simulink model "exercise5s"  (R2025b)
settings: Solver=VariableStepAuto  StartTime=0.0  StopTime=0.01  RelTol=1e-3
values from neighbouring files (symbols this model uses):
  cm = 23.4e-3    (= 0.0234)    [exercise5.m]
  D = 0.4191e-5    (= 4.191e-06)    [exercise5.m]
  J = 0.23e-6    (= 2.3e-07)    [exercise5.m]
  L = 0.23e-3    (= 0.00023)    [exercise5.m]
  R = 2.4    [exercise5.m]
libraries: cstblocks x2
settings Model: Creator=Lenovo  LastModifiedBy=Lenovo

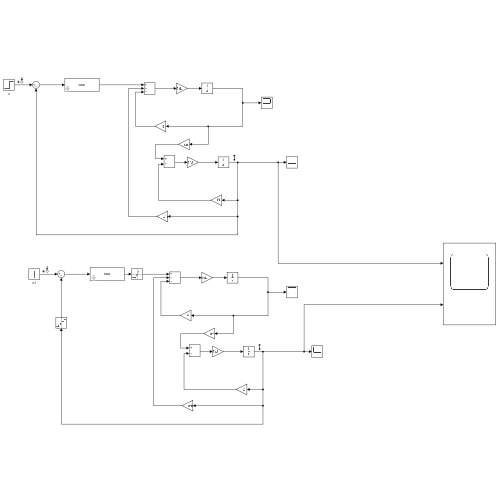
[thumbnail: Simulink's stored preview of the top-level diagram]
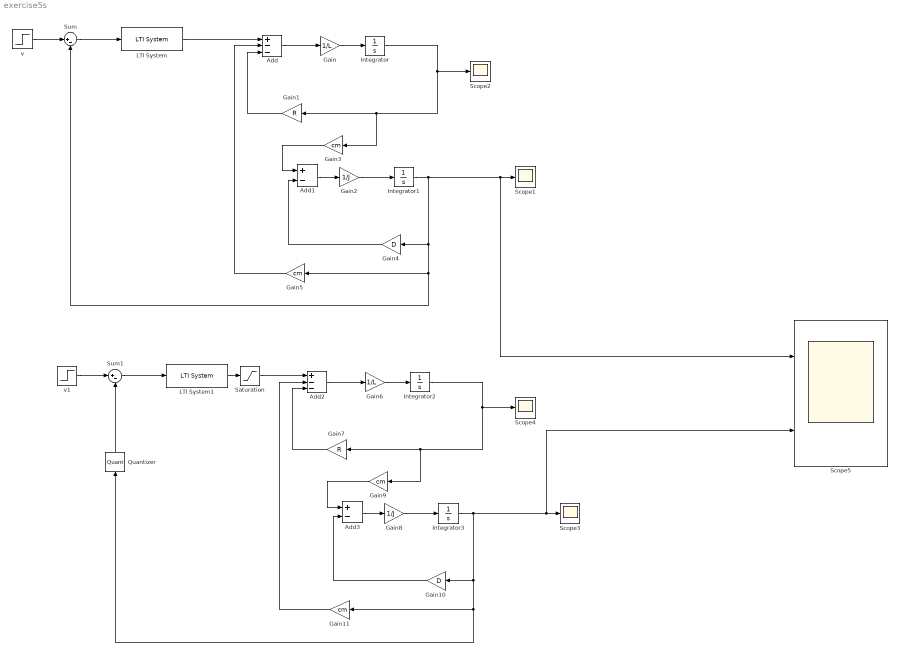
== system exercise5s ==
  Add : Sum  Inputs=+--
  Add1 : Sum  Inputs=+-
  Add2 : Sum  Inputs=+--
  Add3 : Sum  Inputs=+-
  Gain : Gain  Gain=1/L
  Gain1 : Gain  Gain=R
  Gain10 : Gain  Gain=D
  Gain{3,5,9,11} (4 alike) : Gain  Gain=cm
  Gain2 : Gain  Gain=1/J
  Gain4 : Gain  Gain=D
  Gain6 : Gain  Gain=1/L
  Gain7 : Gain  Gain=R
  Gain8 : Gain  Gain=1/J
  Integrator{,1..3} (4 alike) : Integrator
  LTI System : cstblocks/LTI System  sys=cwe  IC=[]  PadeOrder=0
  LTI System1 : cstblocks/LTI System  sys=cwe  IC=[]  PadeOrder=0
  Quantizer : Quantizer  QuantizationInterval=5
  Saturation : Saturate  UpperLimit=12  LowerLimit=-12
  Scope{1..4} (4 alike) : Scope
      Scope1 settings: ActiveDisplayYMinimum=-1  ActiveDisplayYMaximum=1  DataLoggingVariableName=cx
      Scope2 settings: ActiveDisplayYMinimum=-1  ActiveDisplayYMaximum=1  DataLoggingVariableName=cx1
      Scope3 settings: ActiveDisplayYMinimum=-1  ActiveDisplayYMaximum=1  DataLoggingVariableName=cx2
      Scope4 settings: ActiveDisplayYMinimum=-1  ActiveDisplayYMaximum=1  DataLoggingVariableName=cx3
  Scope5 : Scope  NumInputPorts=2
      settings: ActiveDisplayYMinimum=-39.982641044821122  ActiveDisplayYMaximum=359.84376940339018  DataLoggingVariableName=ex5
  Sum : Sum  Inputs=|+-
  Sum1 : Sum  Inputs=|+-
  v : Step  Time=0.001  After=3000*2*3.14/60  SampleTime=0
  v1 : Step  Time=0.001  After=3000*2*3.14/60  SampleTime=0
  wires:
  Gain/1 -> Integrator/1
  Gain3/1 -> Add1/1
  Gain4/1 -> Add1/2
  Add1/1 -> Gain2/1
  Integrator/1 -> Scope2/1, Gain3/1, Gain1/1
  Gain5/1 -> Add/2
  Gain2/1 -> Integrator1/1
  Gain1/1 -> Add/3
  Add/1 -> Gain/1
  Integrator1/1 -> Gain5/1, Sum/2, Gain4/1, Scope5/1, Scope1/1
  Sum/1 -> LTI System/1
  LTI System/1 -> Add/1
  v/1 -> Sum/1
  LTI System1/1 -> Saturation/1
  v1/1 -> Sum1/1
  Sum1/1 -> LTI System1/1
  Add3/1 -> Gain8/1
  Gain7/1 -> Add2/3
  Gain9/1 -> Add3/1
  Gain8/1 -> Integrator3/1
  Integrator3/1 -> Gain11/1, Quantizer/1, Gain10/1, Scope5/2, Scope3/1
  Gain11/1 -> Add2/2
  Gain6/1 -> Integrator2/1
  Integrator2/1 -> Scope4/1, Gain9/1, Gain7/1
  Gain10/1 -> Add3/2
  Add2/1 -> Gain6/1
  Saturation/1 -> Add2/1
  Quantizer/1 -> Sum1/2
